simulink model "SigProcessFinished"  (R2022b)
settings: configuration reference "TmVcThermal_Configuration_sub" (kept outside this file)
undefined symbols (not defined in the file): cClCddAdc_D_u16ADNum, cClCddAdc_D_u8FilterType, cClCddAdc_D_u8RawValueNum
libraries: simulink x23
(part 1 of 2)
settings Model: PacingRate=0.500000  Creator=blue.ge  LastModifiedBy=blue.ge
settings ConfigSetRef: SourceName=TmVcThermal_Configuration_sub  SourceLocation=Base Workspace

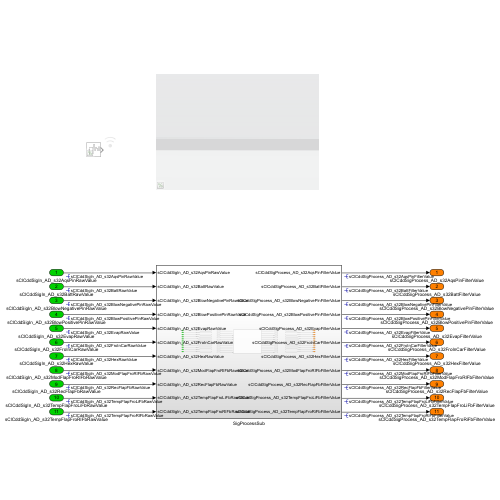
[thumbnail: Simulink's stored preview of the top-level diagram]
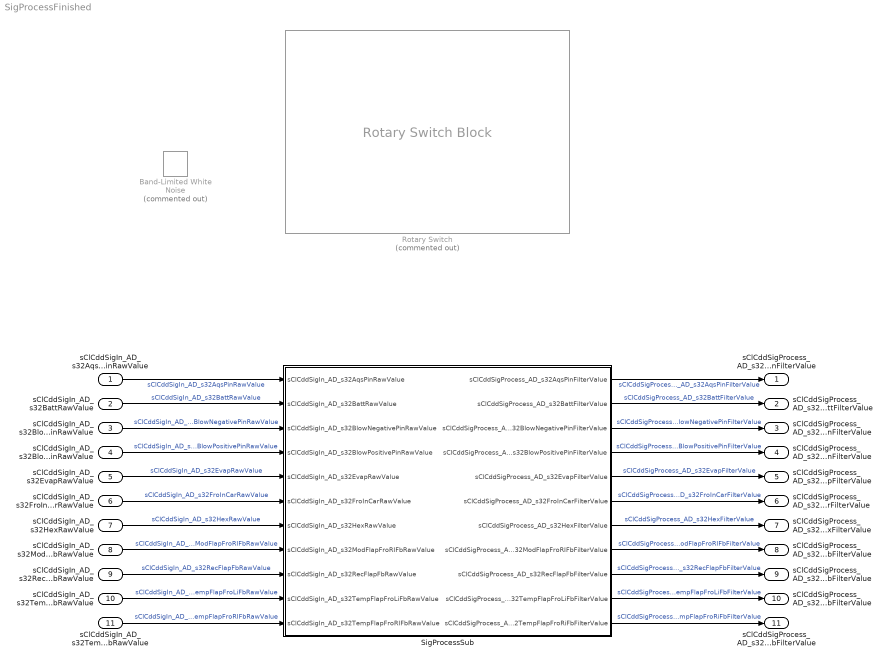
== system SigProcessFinished ==
  sClCddSigIn_AD_s32AqsPinRawValue : Inport  OutDataTypeStr=single
  sClCddSigIn_AD_s32BattRawValue : Inport  Port=2  OutDataTypeStr=single
  sClCddSigIn_AD_s32BlowNegativePinRawValue : Inport  Port=3  OutDataTypeStr=single
  sClCddSigIn_AD_s32BlowPositivePinRawValue : Inport  Port=4  OutDataTypeStr=single
  sClCddSigIn_AD_s32EvapRawValue : Inport  Port=5  OutDataTypeStr=single
  sClCddSigIn_AD_s32FroInCarRawValue : Inport  Port=6  OutDataTypeStr=single
  sClCddSigIn_AD_s32HexRawValue : Inport  Port=7  OutDataTypeStr=single
  sClCddSigIn_AD_s32ModFlapFroRIFbRawValue : Inport  Port=8  OutDataTypeStr=single
  sClCddSigIn_AD_s32RecFlapFbRawValue : Inport  Port=9  OutDataTypeStr=single
  sClCddSigIn_AD_s32TempFlapFroLiFbRawValue : Inport  Port=10  OutDataTypeStr=single
  sClCddSigIn_AD_s32TempFlapFroRIFbRawValue : Inport  Port=11  OutDataTypeStr=single
  Band-Limited White Noise : simulink/Sources/Band-Limited White Noise  Commented=on  Cov=[0.1]  Ts=0.1  seed=[23341]
  Rotary Switch : RotarySwitchBlock  Commented=on
      settings: Values={{'No Filter', 'AvgSortMid', 'AvgSortWithoutEdge', 'AvgSimple', 'AvgQuick'}, [0 1 2 3 4]}
  SigProcessSub : Subsystem
  sClCddSigProcess_AD_s32AqsPinFilterValue : Outport  OutDataTypeStr=single
  sClCddSigProcess_AD_s32BattFilterValue : Outport  Port=2  OutDataTypeStr=single
  sClCddSigProcess_AD_s32BlowNegativePinFilterValue : Outport  Port=3  OutDataTypeStr=single
  sClCddSigProcess_AD_s32BlowPositivePinFilterValue : Outport  Port=4  OutDataTypeStr=single
  sClCddSigProcess_AD_s32EvapFilterValue : Outport  Port=5  OutDataTypeStr=single
  sClCddSigProcess_AD_s32FroInCarFilterValue : Outport  Port=6  OutDataTypeStr=single
  sClCddSigProcess_AD_s32HexFilterValue : Outport  Port=7  OutDataTypeStr=single
  sClCddSigProcess_AD_s32ModFlapFroRIFbFilterValue : Outport  Port=8  OutDataTypeStr=single
  sClCddSigProcess_AD_s32RecFlapFbFilterValue : Outport  Port=9  OutDataTypeStr=single
  sClCddSigProcess_AD_s32TempFlapFroLiFbFilterValue : Outport  Port=10  OutDataTypeStr=single
  sClCddSigProcess_AD_s32TempFlapFroRiFbFilterValue : Outport  Port=11  OutDataTypeStr=single
  wires:
  sClCddSigIn_AD_s32AqsPinRawValue/1 -> SigProcessSub/1(sClCddSigIn_AD_s32AqsPinRawValue)  "sClCddSigIn_AD_s32AqsPinRawValue"
  sClCddSigIn_AD_s32BattRawValue/1 -> SigProcessSub/2(sClCddSigIn_AD_s32BattRawValue)  "sClCddSigIn_AD_s32BattRawValue"
  sClCddSigIn_AD_s32BlowNegativePinRawValue/1 -> SigProcessSub/3(sClCddSigIn_AD_s32BlowNegativePinRawValue)  "sClCddSigIn_AD_s32BlowNegativePinRawValue"
  sClCddSigIn_AD_s32BlowPositivePinRawValue/1 -> SigProcessSub/4(sClCddSigIn_AD_s32BlowPositivePinRawValue)  "sClCddSigIn_AD_s32BlowPositivePinRawValue"
  sClCddSigIn_AD_s32EvapRawValue/1 -> SigProcessSub/5(sClCddSigIn_AD_s32EvapRawValue)  "sClCddSigIn_AD_s32EvapRawValue"
  sClCddSigIn_AD_s32FroInCarRawValue/1 -> SigProcessSub/6(sClCddSigIn_AD_s32FroInCarRawValue)  "sClCddSigIn_AD_s32FroInCarRawValue"
  sClCddSigIn_AD_s32HexRawValue/1 -> SigProcessSub/7(sClCddSigIn_AD_s32HexRawValue)  "sClCddSigIn_AD_s32HexRawValue"
  sClCddSigIn_AD_s32ModFlapFroRIFbRawValue/1 -> SigProcessSub/8(sClCddSigIn_AD_s32ModFlapFroRIFbRawValue)  "sClCddSigIn_AD_s32ModFlapFroRIFbRawValue"
  sClCddSigIn_AD_s32RecFlapFbRawValue/1 -> SigProcessSub/9(sClCddSigIn_AD_s32RecFlapFbRawValue)  "sClCddSigIn_AD_s32RecFlapFbRawValue"
  sClCddSigIn_AD_s32TempFlapFroLiFbRawValue/1 -> SigProcessSub/10(sClCddSigIn_AD_s32TempFlapFroLiFbRawValue)  "sClCddSigIn_AD_s32TempFlapFroLiFbRawValue"
  sClCddSigIn_AD_s32TempFlapFroRIFbRawValue/1 -> SigProcessSub/11(sClCddSigIn_AD_s32TempFlapFroRIFbRawValue)  "sClCddSigIn_AD_s32TempFlapFroRIFbRawValue"
  SigProcessSub/1(sClCddSigProcess_AD_s32AqsPinFilterValue) -> sClCddSigProcess_AD_s32AqsPinFilterValue/1  "sClCddSigProcess_AD_s32AqsPinFilterValue"
  SigProcessSub/2(sClCddSigProcess_AD_s32BattFilterValue) -> sClCddSigProcess_AD_s32BattFilterValue/1  "sClCddSigProcess_AD_s32BattFilterValue"
  SigProcessSub/3(sClCddSigProcess_AD_s32BlowNegativePinFilterValue) -> sClCddSigProcess_AD_s32BlowNegativePinFilterValue/1  "sClCddSigProcess_AD_s32BlowNegativePinFilterValue"
  SigProcessSub/4(sClCddSigProcess_AD_s32BlowPositivePinFilterValue) -> sClCddSigProcess_AD_s32BlowPositivePinFilterValue/1  "sClCddSigProcess_AD_s32BlowPositivePinFilterValue"
  SigProcessSub/5(sClCddSigProcess_AD_s32EvapFilterValue) -> sClCddSigProcess_AD_s32EvapFilterValue/1  "sClCddSigProcess_AD_s32EvapFilterValue"
  SigProcessSub/6(sClCddSigProcess_AD_s32FroInCarFilterValue) -> sClCddSigProcess_AD_s32FroInCarFilterValue/1  "sClCddSigProcess_AD_s32FroInCarFilterValue"
  SigProcessSub/7(sClCddSigProcess_AD_s32HexFilterValue) -> sClCddSigProcess_AD_s32HexFilterValue/1  "sClCddSigProcess_AD_s32HexFilterValue"
  SigProcessSub/8(sClCddSigProcess_AD_s32ModFlapFroRIFbFilterValue) -> sClCddSigProcess_AD_s32ModFlapFroRIFbFilterValue/1  "sClCddSigProcess_AD_s32ModFlapFroRIFbFilterValue"
  SigProcessSub/9(sClCddSigProcess_AD_s32RecFlapFbFilterValue) -> sClCddSigProcess_AD_s32RecFlapFbFilterValue/1  "sClCddSigProcess_AD_s32RecFlapFbFilterValue"
  SigProcessSub/10(sClCddSigProcess_AD_s32TempFlapFroLiFbFilterValue) -> sClCddSigProcess_AD_s32TempFlapFroLiFbFilterValue/1  "sClCddSigProcess_AD_s32TempFlapFroLiFbFilterValue"
  SigProcessSub/11(sClCddSigProcess_AD_s32TempFlapFroRiFbFilterValue) -> sClCddSigProcess_AD_s32TempFlapFroRiFbFilterValue/1  "sClCddSigProcess_AD_s32TempFlapFroRiFbFilterValue"

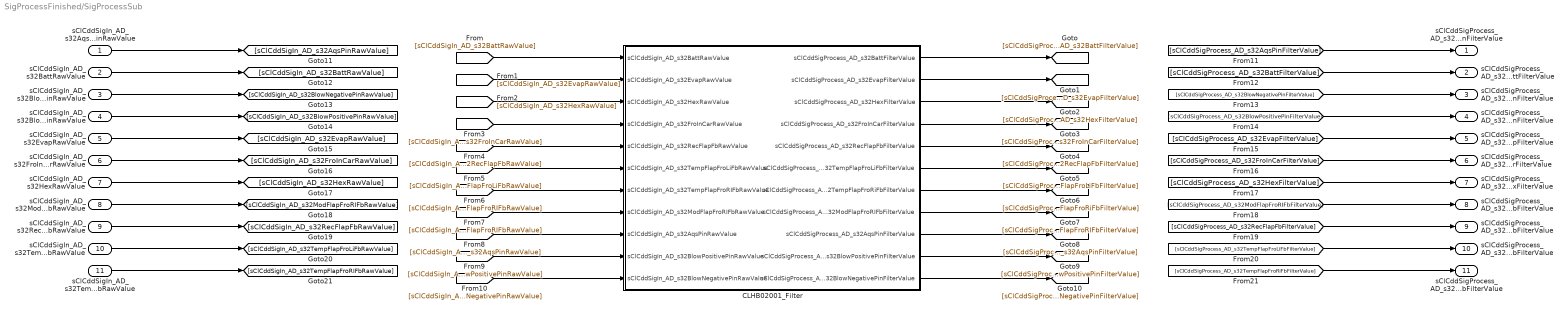
== system SigProcessFinished/SigProcessSub ==
  sClCddSigIn_AD_s32AqsPinRawValue : Inport  OutDataTypeStr=single
  sClCddSigIn_AD_s32BattRawValue : Inport  Port=2  OutDataTypeStr=single
  sClCddSigIn_AD_s32BlowNegativePinRawValue : Inport  Port=3  OutDataTypeStr=single
  sClCddSigIn_AD_s32BlowPositivePinRawValue : Inport  Port=4  OutDataTypeStr=single
  sClCddSigIn_AD_s32EvapRawValue : Inport  Port=5  OutDataTypeStr=single
  sClCddSigIn_AD_s32FroInCarRawValue : Inport  Port=6  OutDataTypeStr=single
  sClCddSigIn_AD_s32HexRawValue : Inport  Port=7  OutDataTypeStr=single
  sClCddSigIn_AD_s32ModFlapFroRIFbRawValue : Inport  Port=8  OutDataTypeStr=single
  sClCddSigIn_AD_s32RecFlapFbRawValue : Inport  Port=9  OutDataTypeStr=single
  sClCddSigIn_AD_s32TempFlapFroLiFbRawValue : Inport  Port=10  OutDataTypeStr=single
  sClCddSigIn_AD_s32TempFlapFroRIFbRawValue : Inport  Port=11  OutDataTypeStr=single
  CLHB02001_Filter : Subsystem
  sClCddSigProcess_AD_s32AqsPinFilterValue : Outport  OutDataTypeStr=single
  sClCddSigProcess_AD_s32BattFilterValue : Outport  Port=2  OutDataTypeStr=single
  sClCddSigProcess_AD_s32BlowNegativePinFilterValue : Outport  Port=3  OutDataTypeStr=single
  sClCddSigProcess_AD_s32BlowPositivePinFilterValue : Outport  Port=4  OutDataTypeStr=single
  sClCddSigProcess_AD_s32EvapFilterValue : Outport  Port=5  OutDataTypeStr=single
  sClCddSigProcess_AD_s32FroInCarFilterValue : Outport  Port=6  OutDataTypeStr=single
  sClCddSigProcess_AD_s32HexFilterValue : Outport  Port=7  OutDataTypeStr=single
  sClCddSigProcess_AD_s32ModFlapFroRIFbFilterValue : Outport  Port=8  OutDataTypeStr=single
  sClCddSigProcess_AD_s32RecFlapFbFilterValue : Outport  Port=9  OutDataTypeStr=single
  sClCddSigProcess_AD_s32TempFlapFroLiFbFilterValue : Outport  Port=10  OutDataTypeStr=single
  sClCddSigProcess_AD_s32TempFlapFroRiFbFilterValue : Outport  Port=11  OutDataTypeStr=single
  wires:
  [sClCddSigIn_AD_s32BattRawValue] -> CLHB02001_Filter/1(sClCddSigIn_AD_s32BattRawValue)
  [sClCddSigIn_AD_s32EvapRawValue] -> CLHB02001_Filter/2(sClCddSigIn_AD_s32EvapRawValue)
  [sClCddSigIn_AD_s32HexRawValue] -> CLHB02001_Filter/3(sClCddSigIn_AD_s32HexRawValue)
  [sClCddSigIn_AD_s32FroInCarRawValue] -> CLHB02001_Filter/4(sClCddSigIn_AD_s32FroInCarRawValue)
  [sClCddSigIn_AD_s32RecFlapFbRawValue] -> CLHB02001_Filter/5(sClCddSigIn_AD_s32RecFlapFbRawValue)
  [sClCddSigIn_AD_s32TempFlapFroLiFbRawValue] -> CLHB02001_Filter/6(sClCddSigIn_AD_s32TempFlapFroLiFbRawValue)
  [sClCddSigIn_AD_s32TempFlapFroRIFbRawValue] -> CLHB02001_Filter/7(sClCddSigIn_AD_s32TempFlapFroRIFbRawValue)
  [sClCddSigIn_AD_s32ModFlapFroRIFbRawValue] -> CLHB02001_Filter/8(sClCddSigIn_AD_s32ModFlapFroRIFbRawValue)
  [sClCddSigIn_AD_s32AqsPinRawValue] -> CLHB02001_Filter/9(sClCddSigIn_AD_s32AqsPinRawValue)
  [sClCddSigIn_AD_s32BlowPositivePinRawValue] -> CLHB02001_Filter/10(sClCddSigIn_AD_s32BlowPositivePinRawValue)
  [sClCddSigIn_AD_s32BlowNegativePinRawValue] -> CLHB02001_Filter/11(sClCddSigIn_AD_s32BlowNegativePinRawValue)
  CLHB02001_Filter/1(sClCddSigProcess_AD_s32BattFilterValue) -> [sClCddSigProcess_AD_s32BattFilterValue]
  CLHB02001_Filter/2(sClCddSigProcess_AD_s32EvapFilterValue) -> [sClCddSigProcess_AD_s32EvapFilterValue]
  CLHB02001_Filter/3(sClCddSigProcess_AD_s32HexFilterValue) -> [sClCddSigProcess_AD_s32HexFilterValue]
  CLHB02001_Filter/4(sClCddSigProcess_AD_s32FroInCarFilterValue) -> [sClCddSigProcess_AD_s32FroInCarFilterValue]
  CLHB02001_Filter/5(sClCddSigProcess_AD_s32RecFlapFbFilterValue) -> [sClCddSigProcess_AD_s32RecFlapFbFilterValue]
  CLHB02001_Filter/6(sClCddSigProcess_AD_s32TempFlapFroLiFbFilterValue) -> [sClCddSigProcess_AD_s32TempFlapFroLiFbFilterValue]
  CLHB02001_Filter/7(sClCddSigProcess_AD_s32TempFlapFroRiFbFilterValue) -> [sClCddSigProcess_AD_s32TempFlapFroRiFbFilterValue]
  CLHB02001_Filter/8(sClCddSigProcess_AD_s32ModFlapFroRIFbFilterValue) -> [sClCddSigProcess_AD_s32ModFlapFroRIFbFilterValue]
  CLHB02001_Filter/9(sClCddSigProcess_AD_s32AqsPinFilterValue) -> [sClCddSigProcess_AD_s32AqsPinFilterValue]
  CLHB02001_Filter/10(sClCddSigProcess_AD_s32BlowPositivePinFilterValue) -> [sClCddSigProcess_AD_s32BlowPositivePinFilterValue]
  CLHB02001_Filter/11(sClCddSigProcess_AD_s32BlowNegativePinFilterValue) -> [sClCddSigProcess_AD_s32BlowNegativePinFilterValue]
  sClCddSigIn_AD_s32AqsPinRawValue/1 -> [sClCddSigIn_AD_s32AqsPinRawValue]
  sClCddSigIn_AD_s32BattRawValue/1 -> [sClCddSigIn_AD_s32BattRawValue]
  sClCddSigIn_AD_s32BlowNegativePinRawValue/1 -> [sClCddSigIn_AD_s32BlowNegativePinRawValue]
  sClCddSigIn_AD_s32BlowPositivePinRawValue/1 -> [sClCddSigIn_AD_s32BlowPositivePinRawValue]
  sClCddSigIn_AD_s32EvapRawValue/1 -> [sClCddSigIn_AD_s32EvapRawValue]
  sClCddSigIn_AD_s32FroInCarRawValue/1 -> [sClCddSigIn_AD_s32FroInCarRawValue]
  sClCddSigIn_AD_s32HexRawValue/1 -> [sClCddSigIn_AD_s32HexRawValue]
  sClCddSigIn_AD_s32ModFlapFroRIFbRawValue/1 -> [sClCddSigIn_AD_s32ModFlapFroRIFbRawValue]
  sClCddSigIn_AD_s32RecFlapFbRawValue/1 -> [sClCddSigIn_AD_s32RecFlapFbRawValue]
  sClCddSigIn_AD_s32TempFlapFroLiFbRawValue/1 -> [sClCddSigIn_AD_s32TempFlapFroLiFbRawValue]
  sClCddSigIn_AD_s32TempFlapFroRIFbRawValue/1 -> [sClCddSigIn_AD_s32TempFlapFroRIFbRawValue]
  [sClCddSigProcess_AD_s32AqsPinFilterValue] -> sClCddSigProcess_AD_s32AqsPinFilterValue/1
  [sClCddSigProcess_AD_s32BattFilterValue] -> sClCddSigProcess_AD_s32BattFilterValue/1
  [sClCddSigProcess_AD_s32BlowNegativePinFilterValue] -> sClCddSigProcess_AD_s32BlowNegativePinFilterValue/1
  [sClCddSigProcess_AD_s32BlowPositivePinFilterValue] -> sClCddSigProcess_AD_s32BlowPositivePinFilterValue/1
  [sClCddSigProcess_AD_s32EvapFilterValue] -> sClCddSigProcess_AD_s32EvapFilterValue/1
  [sClCddSigProcess_AD_s32FroInCarFilterValue] -> sClCddSigProcess_AD_s32FroInCarFilterValue/1
  [sClCddSigProcess_AD_s32HexFilterValue] -> sClCddSigProcess_AD_s32HexFilterValue/1
  [sClCddSigProcess_AD_s32ModFlapFroRIFbFilterValue] -> sClCddSigProcess_AD_s32ModFlapFroRIFbFilterValue/1
  [sClCddSigProcess_AD_s32RecFlapFbFilterValue] -> sClCddSigProcess_AD_s32RecFlapFbFilterValue/1
  [sClCddSigProcess_AD_s32TempFlapFroLiFbFilterValue] -> sClCddSigProcess_AD_s32TempFlapFroLiFbFilterValue/1
  [sClCddSigProcess_AD_s32TempFlapFroRiFbFilterValue] -> sClCddSigProcess_AD_s32TempFlapFroRiFbFilterValue/1

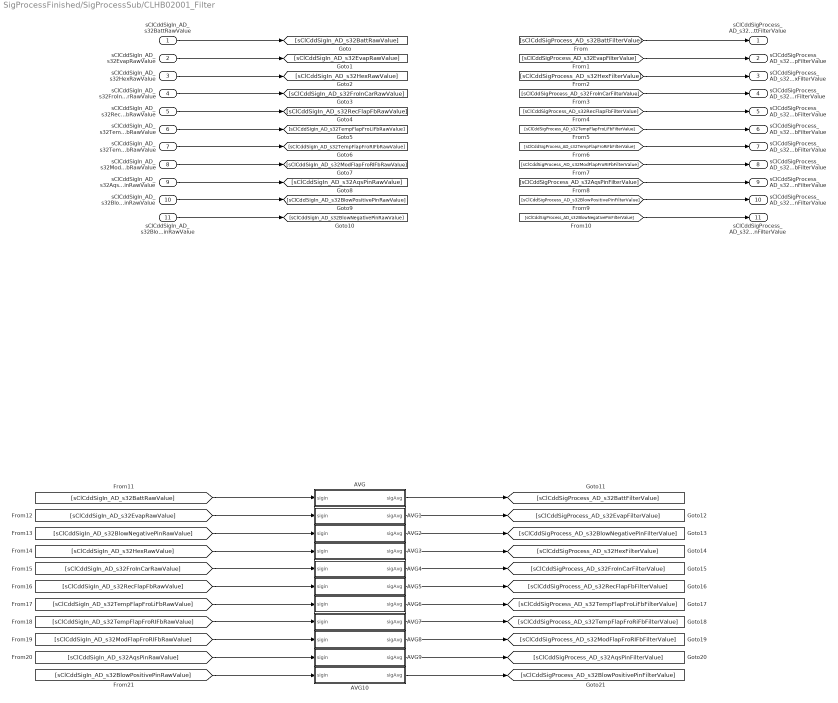
== system SigProcessFinished/SigProcessSub/CLHB02001_Filter ==
  sClCddSigIn_AD_s32BattRawValue : Inport  OutDataTypeStr=single
  sClCddSigIn_AD_s32EvapRawValue : Inport  Port=2  OutDataTypeStr=single
  sClCddSigIn_AD_s32HexRawValue : Inport  Port=3  OutDataTypeStr=single
  sClCddSigIn_AD_s32FroInCarRawValue : Inport  Port=4  OutDataTypeStr=single
  sClCddSigIn_AD_s32RecFlapFbRawValue : Inport  Port=5  OutDataTypeStr=single
  sClCddSigIn_AD_s32TempFlapFroLiFbRawValue : Inport  Port=6  OutDataTypeStr=single
  sClCddSigIn_AD_s32TempFlapFroRIFbRawValue : Inport  Port=7  OutDataTypeStr=single
  sClCddSigIn_AD_s32ModFlapFroRIFbRawValue : Inport  Port=8  OutDataTypeStr=single
  sClCddSigIn_AD_s32AqsPinRawValue : Inport  Port=9  OutDataTypeStr=single
  sClCddSigIn_AD_s32BlowPositivePinRawValue : Inport  Port=10  OutDataTypeStr=single
  sClCddSigIn_AD_s32BlowNegativePinRawValue : Inport  Port=11  OutDataTypeStr=single
  AVG : Subsystem
  AVG1 : Subsystem
  AVG10 : Subsystem
  AVG2 : Subsystem
  AVG3 : Subsystem
  AVG4 : Subsystem
  AVG5 : Subsystem
  AVG6 : Subsystem
  AVG7 : Subsystem
  AVG8 : Subsystem
  AVG9 : Subsystem
  sClCddSigProcess_AD_s32BattFilterValue : Outport  OutDataTypeStr=single
  sClCddSigProcess_AD_s32EvapFilterValue : Outport  Port=2  OutDataTypeStr=single
  sClCddSigProcess_AD_s32HexFilterValue : Outport  Port=3  OutDataTypeStr=single
  sClCddSigProcess_AD_s32FroInCarFilterValue : Outport  Port=4  OutDataTypeStr=single
  sClCddSigProcess_AD_s32RecFlapFbFilterValue : Outport  Port=5  OutDataTypeStr=single
  sClCddSigProcess_AD_s32TempFlapFroLiFbFilterValue : Outport  Port=6  OutDataTypeStr=single
  sClCddSigProcess_AD_s32TempFlapFroRiFbFilterValue : Outport  Port=7  OutDataTypeStr=single
  sClCddSigProcess_AD_s32ModFlapFroRIFbFilterValue : Outport  Port=8  OutDataTypeStr=single
  sClCddSigProcess_AD_s32AqsPinFilterValue : Outport  Port=9  OutDataTypeStr=single
  sClCddSigProcess_AD_s32BlowPositivePinFilterValue : Outport  Port=10  OutDataTypeStr=single
  sClCddSigProcess_AD_s32BlowNegativePinFilterValue : Outport  Port=11  OutDataTypeStr=single
  wires:
  sClCddSigIn_AD_s32BattRawValue/1 -> [sClCddSigIn_AD_s32BattRawValue]
  sClCddSigIn_AD_s32EvapRawValue/1 -> [sClCddSigIn_AD_s32EvapRawValue]
  sClCddSigIn_AD_s32HexRawValue/1 -> [sClCddSigIn_AD_s32HexRawValue]
  sClCddSigIn_AD_s32FroInCarRawValue/1 -> [sClCddSigIn_AD_s32FroInCarRawValue]
  sClCddSigIn_AD_s32RecFlapFbRawValue/1 -> [sClCddSigIn_AD_s32RecFlapFbRawValue]
  sClCddSigIn_AD_s32TempFlapFroLiFbRawValue/1 -> [sClCddSigIn_AD_s32TempFlapFroLiFbRawValue]
  sClCddSigIn_AD_s32TempFlapFroRIFbRawValue/1 -> [sClCddSigIn_AD_s32TempFlapFroRIFbRawValue]
  sClCddSigIn_AD_s32ModFlapFroRIFbRawValue/1 -> [sClCddSigIn_AD_s32ModFlapFroRIFbRawValue]
  sClCddSigIn_AD_s32AqsPinRawValue/1 -> [sClCddSigIn_AD_s32AqsPinRawValue]
  sClCddSigIn_AD_s32BlowPositivePinRawValue/1 -> [sClCddSigIn_AD_s32BlowPositivePinRawValue]
  sClCddSigIn_AD_s32BlowNegativePinRawValue/1 -> [sClCddSigIn_AD_s32BlowNegativePinRawValue]
  [sClCddSigProcess_AD_s32BattFilterValue] -> sClCddSigProcess_AD_s32BattFilterValue/1
  [sClCddSigProcess_AD_s32EvapFilterValue] -> sClCddSigProcess_AD_s32EvapFilterValue/1
  [sClCddSigProcess_AD_s32HexFilterValue] -> sClCddSigProcess_AD_s32HexFilterValue/1
  [sClCddSigProcess_AD_s32FroInCarFilterValue] -> sClCddSigProcess_AD_s32FroInCarFilterValue/1
  [sClCddSigProcess_AD_s32RecFlapFbFilterValue] -> sClCddSigProcess_AD_s32RecFlapFbFilterValue/1
  [sClCddSigProcess_AD_s32TempFlapFroLiFbFilterValue] -> sClCddSigProcess_AD_s32TempFlapFroLiFbFilterValue/1
  [sClCddSigProcess_AD_s32TempFlapFroRiFbFilterValue] -> sClCddSigProcess_AD_s32TempFlapFroRiFbFilterValue/1
  [sClCddSigProcess_AD_s32ModFlapFroRIFbFilterValue] -> sClCddSigProcess_AD_s32ModFlapFroRIFbFilterValue/1
  [sClCddSigProcess_AD_s32AqsPinFilterValue] -> sClCddSigProcess_AD_s32AqsPinFilterValue/1
  [sClCddSigProcess_AD_s32BlowPositivePinFilterValue] -> sClCddSigProcess_AD_s32BlowPositivePinFilterValue/1
  [sClCddSigProcess_AD_s32BlowNegativePinFilterValue] -> sClCddSigProcess_AD_s32BlowNegativePinFilterValue/1
  [sClCddSigIn_AD_s32BattRawValue] -> AVG/1(sigin)
  AVG/1(sigAvg) -> [sClCddSigProcess_AD_s32BattFilterValue]
  [sClCddSigIn_AD_s32EvapRawValue] -> AVG1/1(sigin)
  [sClCddSigIn_AD_s32BlowNegativePinRawValue] -> AVG2/1(sigin)
  [sClCddSigIn_AD_s32HexRawValue] -> AVG3/1(sigin)
  [sClCddSigIn_AD_s32FroInCarRawValue] -> AVG4/1(sigin)
  [sClCddSigIn_AD_s32RecFlapFbRawValue] -> AVG5/1(sigin)
  [sClCddSigIn_AD_s32TempFlapFroLiFbRawValue] -> AVG6/1(sigin)
  [sClCddSigIn_AD_s32TempFlapFroRIFbRawValue] -> AVG7/1(sigin)
  [sClCddSigIn_AD_s32ModFlapFroRIFbRawValue] -> AVG8/1(sigin)
  [sClCddSigIn_AD_s32AqsPinRawValue] -> AVG9/1(sigin)
  [sClCddSigIn_AD_s32BlowPositivePinRawValue] -> AVG10/1(sigin)
  AVG1/1(sigAvg) -> [sClCddSigProcess_AD_s32EvapFilterValue]
  AVG2/1(sigAvg) -> [sClCddSigProcess_AD_s32BlowNegativePinFilterValue]
  AVG3/1(sigAvg) -> [sClCddSigProcess_AD_s32HexFilterValue]
  AVG4/1(sigAvg) -> [sClCddSigProcess_AD_s32FroInCarFilterValue]
  AVG5/1(sigAvg) -> [sClCddSigProcess_AD_s32RecFlapFbFilterValue]
  AVG6/1(sigAvg) -> [sClCddSigProcess_AD_s32TempFlapFroLiFbFilterValue]
  AVG7/1(sigAvg) -> [sClCddSigProcess_AD_s32TempFlapFroRiFbFilterValue]
  AVG8/1(sigAvg) -> [sClCddSigProcess_AD_s32ModFlapFroRIFbFilterValue]
  AVG9/1(sigAvg) -> [sClCddSigProcess_AD_s32AqsPinFilterValue]
  AVG10/1(sigAvg) -> [sClCddSigProcess_AD_s32BlowPositivePinFilterValue]

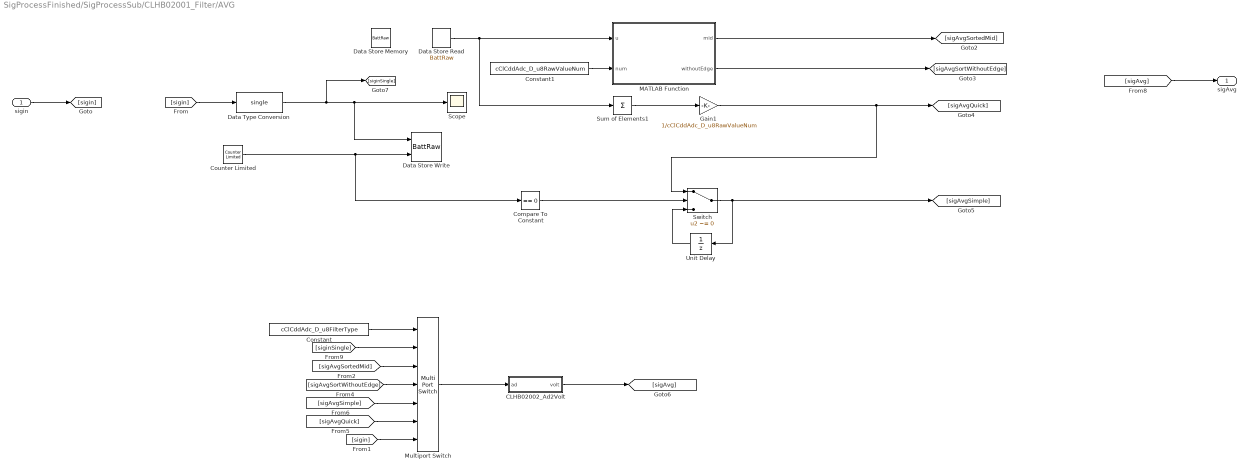
== system SigProcessFinished/SigProcessSub/CLHB02001_Filter/AVG ==
  sigin : Inport
  CLHB02002_Ad2Volt : Subsystem
  Compare To Constant : simulink/Logic and Bit Operations/Compare To Constant  relop===  const=0  OutDataTypeStr=boolean
  Constant : Constant  Value=cClCddAdc_D_u8FilterType  OutDataTypeStr=uint8
  Constant1 : Constant  Value=cClCddAdc_D_u8RawValueNum  OutDataTypeStr=uint8
  Counter Limited : simulink/Sources/Counter Limited  uplimit=cClCddAdc_D_u8RawValueNum-1  tsamp=-1
  Data Store Memory : DataStoreMemory  DataStoreName=BattRaw  ReadBeforeWriteMsg=warning  WriteAfterWriteMsg=warning  WriteAfterReadMsg=warning  ShowAdditionalParam=off  OutDataTypeStr=single  Dimensions=[1 20]
      settings: CopyFcn=set_param(gcbh,'ShowName','off');
  Data Store Read : DataStoreRead  DataStoreName=BattRaw  IndexOptions=Index vector (dialog)  Indices=1  OutputSizes=1
  Data Store Write : DataStoreWrite  DataStoreName=BattRaw  DataStoreElements=BattRaw  EnableIndexing=on  IndexMode=Zero-based  IndexOptions=Index vector (port)  Indices=1  OutputSizes=1
  Data Type Conversion : DataTypeConversion  OutDataTypeStr=single  SaturateOnIntegerOverflow=off  RndMeth=Floor
  Gain1 : Gain  Gain=1/cClCddAdc_D_u8RawValueNum
  MATLAB Function : MATLAB Function  TreatAsAtomicUnit=on
  Multiport Switch : MultiPortSwitch  DataPortOrder=Zero-based contiguous  Inputs=5  DataPortForDefault=Additional data port  zeroidx=on  OutDataTypeStr=single  SaturateOnIntegerOverflow=off  InputSameDT=off
  Scope : Scope
  Sum of Elements1 : Sum  Inputs=+
  Switch : Switch  Criteria=u2 ~= 0  SaturateOnIntegerOverflow=off  InputSameDT=off
  Unit Delay : UnitDelay  SampleTime=-1  HasFrameUpgradeWarning=on
  sigAvg : Outport  OutDataTypeStr=single
  wires:
  Data Store Read/1 -> MATLAB Function/1(u), Sum of Elements1/1
  Sum of Elements1/1 -> Gain1/1
  Compare To Constant/1 -> Switch/2
  Switch/1 -> [sigAvgSimple], Unit Delay/1
  Gain1/1 -> Switch/1, [sigAvgQuick]
  Counter Limited/1 -> Compare To Constant/1, Data Store Write/2
  Data Type Conversion/1 -> [siginSingle], Data Store Write/1, Scope/1
  MATLAB Function/2(withoutEdge) -> [sigAvgSortWithoutEdge]
  Unit Delay/1 -> Switch/3
  MATLAB Function/1(mid) -> [sigAvgSortedMid]
  sigin/1 -> [sigin]
  [sigin] -> Data Type Conversion/1
  [sigin] -> Multiport Switch/7
  Constant/1 -> Multiport Switch/1
  [sigAvgSortedMid] -> Multiport Switch/3
  [sigAvgSortWithoutEdge] -> Multiport Switch/4
  [sigAvgSimple] -> Multiport Switch/5
  [sigAvgQuick] -> Multiport Switch/6
  [siginSingle] -> Multiport Switch/2
  Multiport Switch/1 -> CLHB02002_Ad2Volt/1(ad)
  [sigAvg] -> sigAvg/1
  Constant1/1 -> MATLAB Function/2(num)
  CLHB02002_Ad2Volt/1(volt) -> [sigAvg]

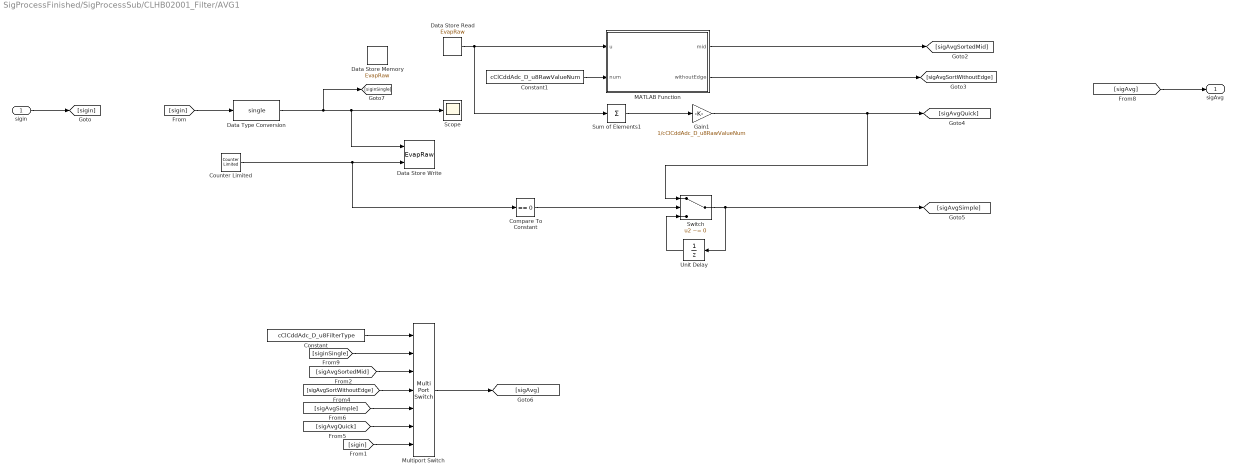
== system SigProcessFinished/SigProcessSub/CLHB02001_Filter/AVG1 ==
  sigin : Inport
  Compare To Constant : simulink/Logic and Bit Operations/Compare To Constant  relop===  const=0  OutDataTypeStr=boolean
  Constant : Constant  Value=cClCddAdc_D_u8FilterType  OutDataTypeStr=uint8
  Constant1 : Constant  Value=cClCddAdc_D_u8RawValueNum  OutDataTypeStr=uint8
  Counter Limited : simulink/Sources/Counter Limited  uplimit=cClCddAdc_D_u8RawValueNum-1  tsamp=-1
  Data Store Memory : DataStoreMemory  DataStoreName=EvapRaw  ReadBeforeWriteMsg=warning  WriteAfterWriteMsg=warning  WriteAfterReadMsg=warning  ShowAdditionalParam=off  OutDataTypeStr=single  Dimensions=[1 20]
      settings: CopyFcn=set_param(gcbh,'ShowName','off');
  Data Store Read : DataStoreRead  DataStoreName=EvapRaw  IndexOptions=Index vector (dialog)  Indices=1  OutputSizes=1
  Data Store Write : DataStoreWrite  DataStoreName=EvapRaw  DataStoreElements=EvapRaw  EnableIndexing=on  IndexMode=Zero-based  IndexOptions=Index vector (port)  Indices=1  OutputSizes=1
  Data Type Conversion : DataTypeConversion  OutDataTypeStr=single  SaturateOnIntegerOverflow=off  RndMeth=Floor
  Gain1 : Gain  Gain=1/cClCddAdc_D_u8RawValueNum
  MATLAB Function : MATLAB Function  TreatAsAtomicUnit=on
  Multiport Switch : MultiPortSwitch  DataPortOrder=Zero-based contiguous  Inputs=5  DataPortForDefault=Additional data port  zeroidx=on  OutDataTypeStr=single  SaturateOnIntegerOverflow=off  InputSameDT=off
  Scope : Scope
  Sum of Elements1 : Sum  Inputs=+
  Switch : Switch  Criteria=u2 ~= 0  SaturateOnIntegerOverflow=off  InputSameDT=off
  Unit Delay : UnitDelay  SampleTime=-1  HasFrameUpgradeWarning=on
  sigAvg : Outport  OutDataTypeStr=single
  wires:
  Constant1/1 -> MATLAB Function/2(num)
  [sigAvg] -> sigAvg/1
  Multiport Switch/1 -> [sigAvg]
  [siginSingle] -> Multiport Switch/2
  [sigAvgQuick] -> Multiport Switch/6
  [sigAvgSimple] -> Multiport Switch/5
  [sigAvgSortWithoutEdge] -> Multiport Switch/4
  [sigAvgSortedMid] -> Multiport Switch/3
  Constant/1 -> Multiport Switch/1
  [sigin] -> Multiport Switch/7
  [sigin] -> Data Type Conversion/1
  sigin/1 -> [sigin]
  MATLAB Function/1(mid) -> [sigAvgSortedMid]
  Unit Delay/1 -> Switch/3
  MATLAB Function/2(withoutEdge) -> [sigAvgSortWithoutEdge]
  Data Type Conversion/1 -> Scope/1, Data Store Write/1, [siginSingle]
  Counter Limited/1 -> Data Store Write/2, Compare To Constant/1
  Gain1/1 -> [sigAvgQuick], Switch/1
  Switch/1 -> Unit Delay/1, [sigAvgSimple]
  Compare To Constant/1 -> Switch/2
  Sum of Elements1/1 -> Gain1/1
  Data Store Read/1 -> Sum of Elements1/1, MATLAB Function/1(u)

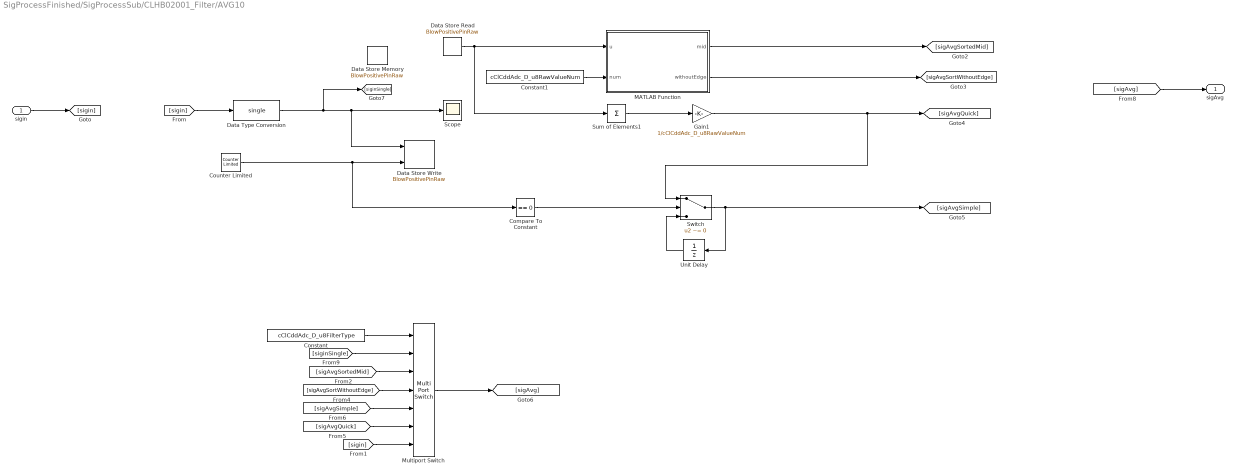
== system SigProcessFinished/SigProcessSub/CLHB02001_Filter/AVG10 ==
  sigin : Inport
  Compare To Constant : simulink/Logic and Bit Operations/Compare To Constant  relop===  const=0  OutDataTypeStr=boolean
  Constant : Constant  Value=cClCddAdc_D_u8FilterType  OutDataTypeStr=uint8
  Constant1 : Constant  Value=cClCddAdc_D_u8RawValueNum  OutDataTypeStr=uint8
  Counter Limited : simulink/Sources/Counter Limited  uplimit=cClCddAdc_D_u8RawValueNum-1  tsamp=-1
  Data Store Memory : DataStoreMemory  DataStoreName=BlowPositivePinRaw  ReadBeforeWriteMsg=warning  WriteAfterWriteMsg=warning  WriteAfterReadMsg=warning  ShowAdditionalParam=off  OutDataTypeStr=single  Dimensions=[1 20]
      settings: CopyFcn=set_param(gcbh,'ShowName','off');
  Data Store Read : DataStoreRead  DataStoreName=BlowPositivePinRaw  IndexOptions=Index vector (dialog)  Indices=1  OutputSizes=1
  Data Store Write : DataStoreWrite  DataStoreName=BlowPositivePinRaw  DataStoreElements=BlowPositivePinRaw  EnableIndexing=on  IndexMode=Zero-based  IndexOptions=Index vector (port)  Indices=1  OutputSizes=1
  Data Type Conversion : DataTypeConversion  OutDataTypeStr=single  SaturateOnIntegerOverflow=off  RndMeth=Floor
  Gain1 : Gain  Gain=1/cClCddAdc_D_u8RawValueNum
  MATLAB Function : MATLAB Function  TreatAsAtomicUnit=on
  Multiport Switch : MultiPortSwitch  DataPortOrder=Zero-based contiguous  Inputs=5  DataPortForDefault=Additional data port  zeroidx=on  OutDataTypeStr=single  SaturateOnIntegerOverflow=off  InputSameDT=off
  Scope : Scope
  Sum of Elements1 : Sum  Inputs=+
  Switch : Switch  Criteria=u2 ~= 0  SaturateOnIntegerOverflow=off  InputSameDT=off
  Unit Delay : UnitDelay  SampleTime=-1  HasFrameUpgradeWarning=on
  sigAvg : Outport  OutDataTypeStr=single
  wires:
  Data Store Read/1 -> MATLAB Function/1(u), Sum of Elements1/1
  Sum of Elements1/1 -> Gain1/1
  Compare To Constant/1 -> Switch/2
  Switch/1 -> [sigAvgSimple], Unit Delay/1
  Gain1/1 -> Switch/1, [sigAvgQuick]
  Counter Limited/1 -> Compare To Constant/1, Data Store Write/2
  Data Type Conversion/1 -> [siginSingle], Data Store Write/1, Scope/1
  MATLAB Function/2(withoutEdge) -> [sigAvgSortWithoutEdge]
  Unit Delay/1 -> Switch/3
  MATLAB Function/1(mid) -> [sigAvgSortedMid]
  sigin/1 -> [sigin]
  [sigin] -> Data Type Conversion/1
  [sigin] -> Multiport Switch/7
  Constant/1 -> Multiport Switch/1
  [sigAvgSortedMid] -> Multiport Switch/3
  [sigAvgSortWithoutEdge] -> Multiport Switch/4
  [sigAvgSimple] -> Multiport Switch/5
  [sigAvgQuick] -> Multiport Switch/6
  [siginSingle] -> Multiport Switch/2
  Multiport Switch/1 -> [sigAvg]
  [sigAvg] -> sigAvg/1
  Constant1/1 -> MATLAB Function/2(num)

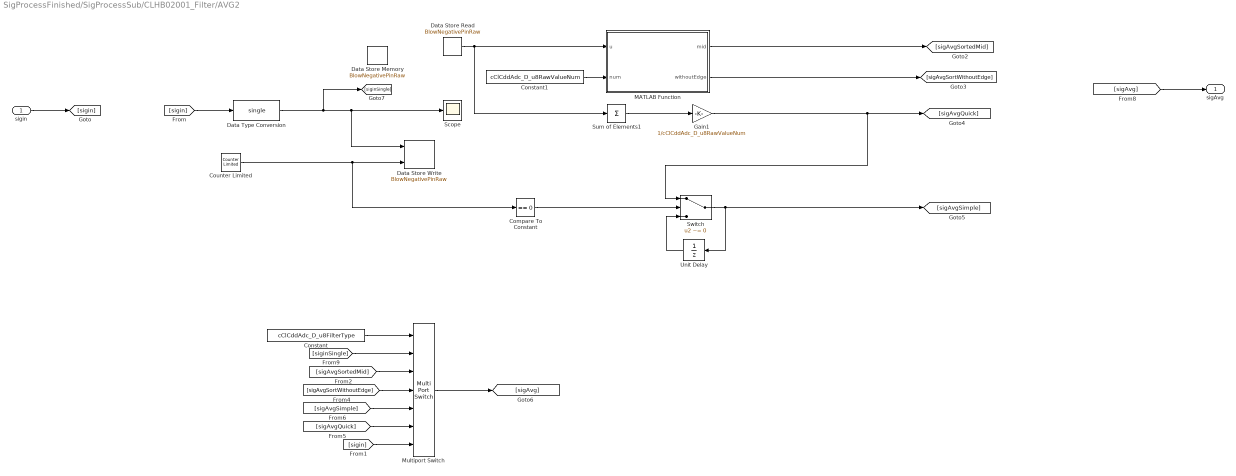
== system SigProcessFinished/SigProcessSub/CLHB02001_Filter/AVG2 ==
  sigin : Inport
  Compare To Constant : simulink/Logic and Bit Operations/Compare To Constant  relop===  const=0  OutDataTypeStr=boolean
  Constant : Constant  Value=cClCddAdc_D_u8FilterType  OutDataTypeStr=uint8
  Constant1 : Constant  Value=cClCddAdc_D_u8RawValueNum  OutDataTypeStr=uint8
  Counter Limited : simulink/Sources/Counter Limited  uplimit=cClCddAdc_D_u8RawValueNum-1  tsamp=-1
  Data Store Memory : DataStoreMemory  DataStoreName=BlowNegativePinRaw  ReadBeforeWriteMsg=warning  WriteAfterWriteMsg=warning  WriteAfterReadMsg=warning  ShowAdditionalParam=off  OutDataTypeStr=single  Dimensions=[1 20]
      settings: CopyFcn=set_param(gcbh,'ShowName','off');
  Data Store Read : DataStoreRead  DataStoreName=BlowNegativePinRaw  IndexOptions=Index vector (dialog)  Indices=1  OutputSizes=1
  Data Store Write : DataStoreWrite  DataStoreName=BlowNegativePinRaw  DataStoreElements=BlowNegativePinRaw  EnableIndexing=on  IndexMode=Zero-based  IndexOptions=Index vector (port)  Indices=1  OutputSizes=1
  Data Type Conversion : DataTypeConversion  OutDataTypeStr=single  SaturateOnIntegerOverflow=off  RndMeth=Floor
  Gain1 : Gain  Gain=1/cClCddAdc_D_u8RawValueNum
  MATLAB Function : MATLAB Function  TreatAsAtomicUnit=on
  Multiport Switch : MultiPortSwitch  DataPortOrder=Zero-based contiguous  Inputs=5  DataPortForDefault=Additional data port  zeroidx=on  OutDataTypeStr=single  SaturateOnIntegerOverflow=off  InputSameDT=off
  Scope : Scope
  Sum of Elements1 : Sum  Inputs=+
  Switch : Switch  Criteria=u2 ~= 0  SaturateOnIntegerOverflow=off  InputSameDT=off
  Unit Delay : UnitDelay  SampleTime=-1  HasFrameUpgradeWarning=on
  sigAvg : Outport  OutDataTypeStr=single
  wires:
  Data Store Read/1 -> MATLAB Function/1(u), Sum of Elements1/1
  Sum of Elements1/1 -> Gain1/1
  Compare To Constant/1 -> Switch/2
  Switch/1 -> [sigAvgSimple], Unit Delay/1
  Gain1/1 -> Switch/1, [sigAvgQuick]
  Counter Limited/1 -> Compare To Constant/1, Data Store Write/2
  Data Type Conversion/1 -> [siginSingle], Data Store Write/1, Scope/1
  MATLAB Function/2(withoutEdge) -> [sigAvgSortWithoutEdge]
  Unit Delay/1 -> Switch/3
  MATLAB Function/1(mid) -> [sigAvgSortedMid]
  sigin/1 -> [sigin]
  [sigin] -> Data Type Conversion/1
  [sigin] -> Multiport Switch/7
  Constant/1 -> Multiport Switch/1
  [sigAvgSortedMid] -> Multiport Switch/3
  [sigAvgSortWithoutEdge] -> Multiport Switch/4
  [sigAvgSimple] -> Multiport Switch/5
  [sigAvgQuick] -> Multiport Switch/6
  [siginSingle] -> Multiport Switch/2
  Multiport Switch/1 -> [sigAvg]
  [sigAvg] -> sigAvg/1
  Constant1/1 -> MATLAB Function/2(num)

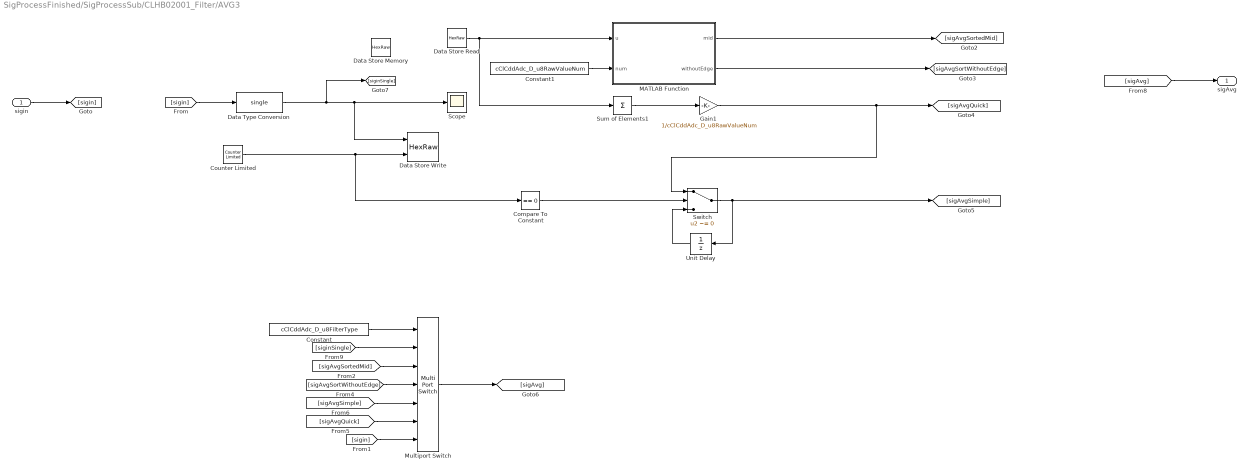
== system SigProcessFinished/SigProcessSub/CLHB02001_Filter/AVG3 ==
  sigin : Inport
  Compare To Constant : simulink/Logic and Bit Operations/Compare To Constant  relop===  const=0  OutDataTypeStr=boolean
  Constant : Constant  Value=cClCddAdc_D_u8FilterType  OutDataTypeStr=uint8
  Constant1 : Constant  Value=cClCddAdc_D_u8RawValueNum  OutDataTypeStr=uint8
  Counter Limited : simulink/Sources/Counter Limited  uplimit=cClCddAdc_D_u8RawValueNum-1  tsamp=-1
  Data Store Memory : DataStoreMemory  DataStoreName=HexRaw  ReadBeforeWriteMsg=warning  WriteAfterWriteMsg=warning  WriteAfterReadMsg=warning  ShowAdditionalParam=off  OutDataTypeStr=single  Dimensions=[1 20]
      settings: CopyFcn=set_param(gcbh,'ShowName','off');
  Data Store Read : DataStoreRead  DataStoreName=HexRaw  IndexOptions=Index vector (dialog)  Indices=1  OutputSizes=1
  Data Store Write : DataStoreWrite  DataStoreName=HexRaw  DataStoreElements=HexRaw  EnableIndexing=on  IndexMode=Zero-based  IndexOptions=Index vector (port)  Indices=1  OutputSizes=1
  Data Type Conversion : DataTypeConversion  OutDataTypeStr=single  SaturateOnIntegerOverflow=off  RndMeth=Floor
  Gain1 : Gain  Gain=1/cClCddAdc_D_u8RawValueNum
  MATLAB Function : MATLAB Function  TreatAsAtomicUnit=on
  Multiport Switch : MultiPortSwitch  DataPortOrder=Zero-based contiguous  Inputs=5  DataPortForDefault=Additional data port  zeroidx=on  OutDataTypeStr=single  SaturateOnIntegerOverflow=off  InputSameDT=off
  Scope : Scope
  Sum of Elements1 : Sum  Inputs=+
  Switch : Switch  Criteria=u2 ~= 0  SaturateOnIntegerOverflow=off  InputSameDT=off
  Unit Delay : UnitDelay  SampleTime=-1  HasFrameUpgradeWarning=on
  sigAvg : Outport  OutDataTypeStr=single
  wires:
  Constant1/1 -> MATLAB Function/2(num)
  [sigAvg] -> sigAvg/1
  Multiport Switch/1 -> [sigAvg]
  [siginSingle] -> Multiport Switch/2
  [sigAvgQuick] -> Multiport Switch/6
  [sigAvgSimple] -> Multiport Switch/5
  [sigAvgSortWithoutEdge] -> Multiport Switch/4
  [sigAvgSortedMid] -> Multiport Switch/3
  Constant/1 -> Multiport Switch/1
  [sigin] -> Multiport Switch/7
  [sigin] -> Data Type Conversion/1
  sigin/1 -> [sigin]
  MATLAB Function/1(mid) -> [sigAvgSortedMid]
  Unit Delay/1 -> Switch/3
  MATLAB Function/2(withoutEdge) -> [sigAvgSortWithoutEdge]
  Data Type Conversion/1 -> Scope/1, Data Store Write/1, [siginSingle]
  Counter Limited/1 -> Data Store Write/2, Compare To Constant/1
  Gain1/1 -> [sigAvgQuick], Switch/1
  Switch/1 -> Unit Delay/1, [sigAvgSimple]
  Compare To Constant/1 -> Switch/2
  Sum of Elements1/1 -> Gain1/1
  Data Store Read/1 -> Sum of Elements1/1, MATLAB Function/1(u)

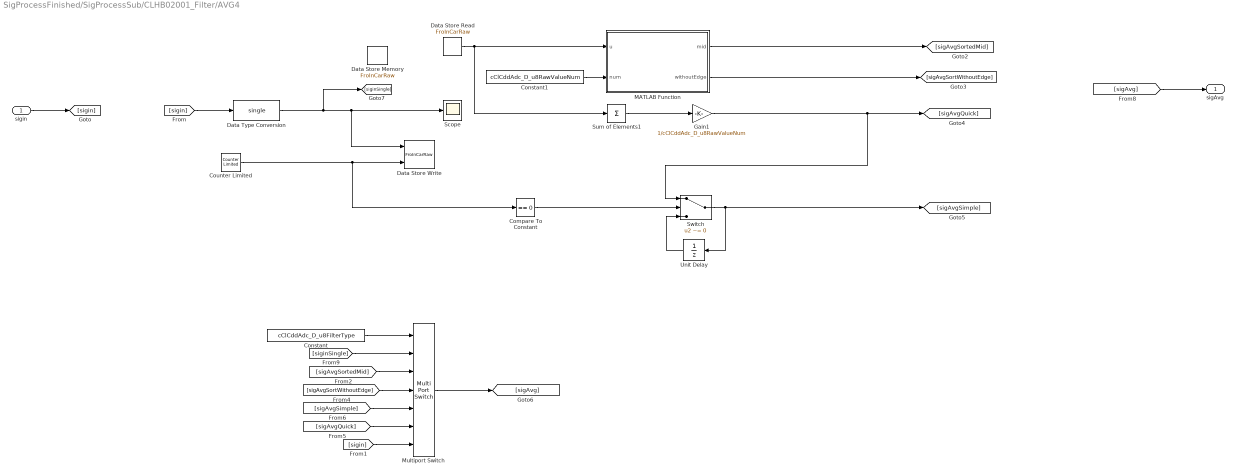
== system SigProcessFinished/SigProcessSub/CLHB02001_Filter/AVG4 ==
  sigin : Inport
  Compare To Constant : simulink/Logic and Bit Operations/Compare To Constant  relop===  const=0  OutDataTypeStr=boolean
  Constant : Constant  Value=cClCddAdc_D_u8FilterType  OutDataTypeStr=uint8
  Constant1 : Constant  Value=cClCddAdc_D_u8RawValueNum  OutDataTypeStr=uint8
  Counter Limited : simulink/Sources/Counter Limited  uplimit=cClCddAdc_D_u8RawValueNum-1  tsamp=-1
  Data Store Memory : DataStoreMemory  DataStoreName=FroInCarRaw  ReadBeforeWriteMsg=warning  WriteAfterWriteMsg=warning  WriteAfterReadMsg=warning  ShowAdditionalParam=off  OutDataTypeStr=single  Dimensions=[1 20]
      settings: CopyFcn=set_param(gcbh,'ShowName','off');
  Data Store Read : DataStoreRead  DataStoreName=FroInCarRaw  IndexOptions=Index vector (dialog)  Indices=1  OutputSizes=1
  Data Store Write : DataStoreWrite  DataStoreName=FroInCarRaw  DataStoreElements=FroInCarRaw  EnableIndexing=on  IndexMode=Zero-based  IndexOptions=Index vector (port)  Indices=1  OutputSizes=1
  Data Type Conversion : DataTypeConversion  OutDataTypeStr=single  SaturateOnIntegerOverflow=off  RndMeth=Floor
  Gain1 : Gain  Gain=1/cClCddAdc_D_u8RawValueNum
  MATLAB Function : MATLAB Function  TreatAsAtomicUnit=on
  Multiport Switch : MultiPortSwitch  DataPortOrder=Zero-based contiguous  Inputs=5  DataPortForDefault=Additional data port  zeroidx=on  OutDataTypeStr=single  SaturateOnIntegerOverflow=off  InputSameDT=off
  Scope : Scope
  Sum of Elements1 : Sum  Inputs=+
  Switch : Switch  Criteria=u2 ~= 0  SaturateOnIntegerOverflow=off  InputSameDT=off
  Unit Delay : UnitDelay  SampleTime=-1  HasFrameUpgradeWarning=on
  sigAvg : Outport  OutDataTypeStr=single
  wires:
  Data Store Read/1 -> MATLAB Function/1(u), Sum of Elements1/1
  Sum of Elements1/1 -> Gain1/1
  Compare To Constant/1 -> Switch/2
  Switch/1 -> [sigAvgSimple], Unit Delay/1
  Gain1/1 -> Switch/1, [sigAvgQuick]
  Counter Limited/1 -> Compare To Constant/1, Data Store Write/2
  Data Type Conversion/1 -> [siginSingle], Data Store Write/1, Scope/1
  MATLAB Function/2(withoutEdge) -> [sigAvgSortWithoutEdge]
  Unit Delay/1 -> Switch/3
  MATLAB Function/1(mid) -> [sigAvgSortedMid]
  sigin/1 -> [sigin]
  [sigin] -> Data Type Conversion/1
  [sigin] -> Multiport Switch/7
  Constant/1 -> Multiport Switch/1
  [sigAvgSortedMid] -> Multiport Switch/3
  [sigAvgSortWithoutEdge] -> Multiport Switch/4
  [sigAvgSimple] -> Multiport Switch/5
  [sigAvgQuick] -> Multiport Switch/6
  [siginSingle] -> Multiport Switch/2
  Multiport Switch/1 -> [sigAvg]
  [sigAvg] -> sigAvg/1
  Constant1/1 -> MATLAB Function/2(num)

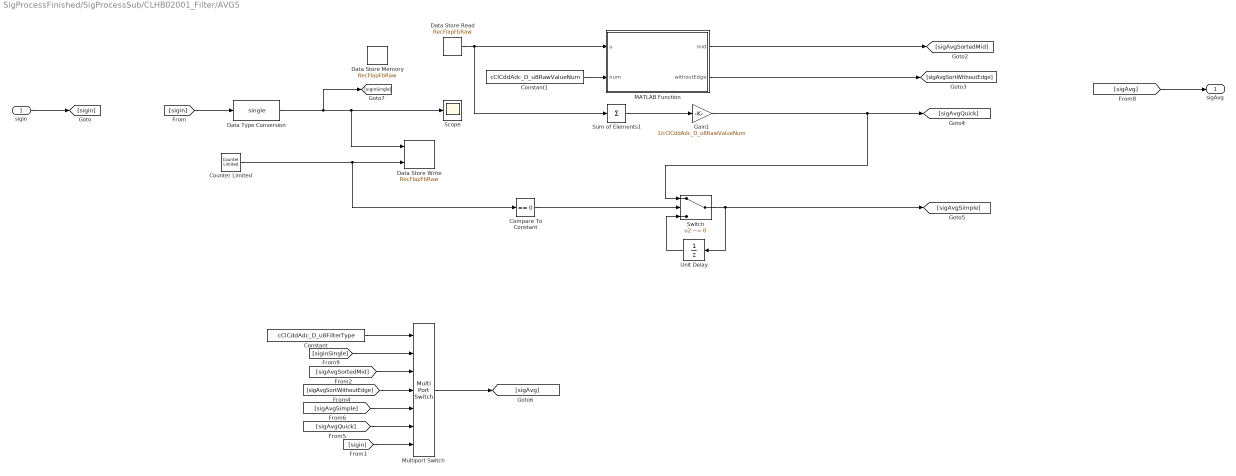
== system SigProcessFinished/SigProcessSub/CLHB02001_Filter/AVG5 ==
  sigin : Inport
  Compare To Constant : simulink/Logic and Bit Operations/Compare To Constant  relop===  const=0  OutDataTypeStr=boolean
  Constant : Constant  Value=cClCddAdc_D_u8FilterType  OutDataTypeStr=uint8
  Constant1 : Constant  Value=cClCddAdc_D_u8RawValueNum  OutDataTypeStr=uint8
  Counter Limited : simulink/Sources/Counter Limited  uplimit=cClCddAdc_D_u8RawValueNum-1  tsamp=-1
  Data Store Memory : DataStoreMemory  DataStoreName=RecFlapFbRaw  ReadBeforeWriteMsg=warning  WriteAfterWriteMsg=warning  WriteAfterReadMsg=warning  ShowAdditionalParam=off  OutDataTypeStr=single  Dimensions=[1 20]
      settings: CopyFcn=set_param(gcbh,'ShowName','off');
  Data Store Read : DataStoreRead  DataStoreName=RecFlapFbRaw  IndexOptions=Index vector (dialog)  Indices=1  OutputSizes=1
  Data Store Write : DataStoreWrite  DataStoreName=RecFlapFbRaw  DataStoreElements=RecFlapFbRaw  EnableIndexing=on  IndexMode=Zero-based  IndexOptions=Index vector (port)  Indices=1  OutputSizes=1
  Data Type Conversion : DataTypeConversion  OutDataTypeStr=single  SaturateOnIntegerOverflow=off  RndMeth=Floor
  Gain1 : Gain  Gain=1/cClCddAdc_D_u8RawValueNum
  MATLAB Function : MATLAB Function  TreatAsAtomicUnit=on
  Multiport Switch : MultiPortSwitch  DataPortOrder=Zero-based contiguous  Inputs=5  DataPortForDefault=Additional data port  zeroidx=on  OutDataTypeStr=single  SaturateOnIntegerOverflow=off  InputSameDT=off
  Scope : Scope
  Sum of Elements1 : Sum  Inputs=+
  Switch : Switch  Criteria=u2 ~= 0  SaturateOnIntegerOverflow=off  InputSameDT=off
  Unit Delay : UnitDelay  SampleTime=-1  HasFrameUpgradeWarning=on
  sigAvg : Outport  OutDataTypeStr=single
  wires:
  Constant1/1 -> MATLAB Function/2(num)
  [sigAvg] -> sigAvg/1
  Multiport Switch/1 -> [sigAvg]
  [siginSingle] -> Multiport Switch/2
  [sigAvgQuick] -> Multiport Switch/6
  [sigAvgSimple] -> Multiport Switch/5
  [sigAvgSortWithoutEdge] -> Multiport Switch/4
  [sigAvgSortedMid] -> Multiport Switch/3
  Constant/1 -> Multiport Switch/1
  [sigin] -> Multiport Switch/7
  [sigin] -> Data Type Conversion/1
  sigin/1 -> [sigin]
  MATLAB Function/1(mid) -> [sigAvgSortedMid]
  Unit Delay/1 -> Switch/3
  MATLAB Function/2(withoutEdge) -> [sigAvgSortWithoutEdge]
  Data Type Conversion/1 -> Scope/1, Data Store Write/1, [siginSingle]
  Counter Limited/1 -> Data Store Write/2, Compare To Constant/1
  Gain1/1 -> [sigAvgQuick], Switch/1
  Switch/1 -> Unit Delay/1, [sigAvgSimple]
  Compare To Constant/1 -> Switch/2
  Sum of Elements1/1 -> Gain1/1
  Data Store Read/1 -> Sum of Elements1/1, MATLAB Function/1(u)

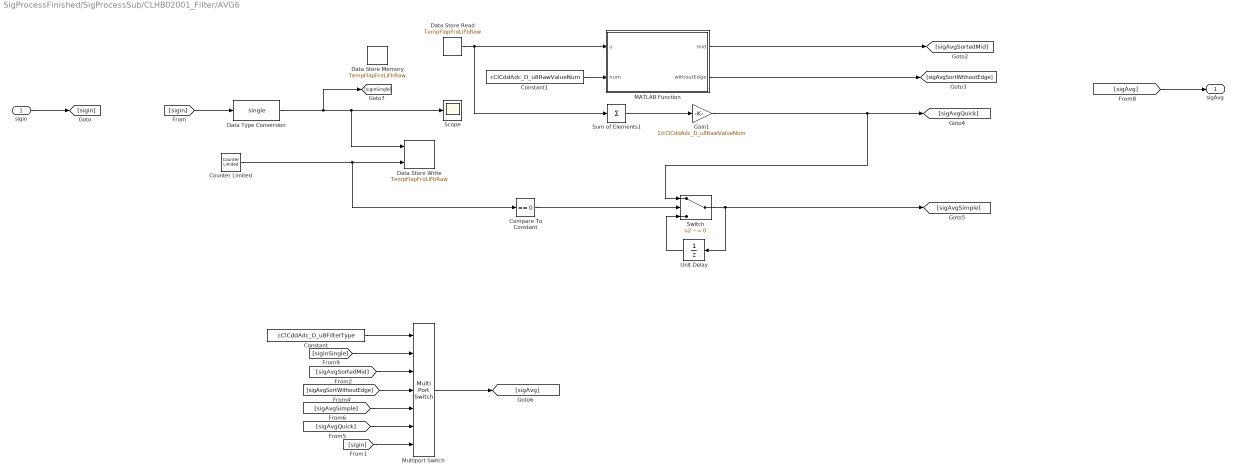
== system SigProcessFinished/SigProcessSub/CLHB02001_Filter/AVG6 ==
  sigin : Inport
  Compare To Constant : simulink/Logic and Bit Operations/Compare To Constant  relop===  const=0  OutDataTypeStr=boolean
  Constant : Constant  Value=cClCddAdc_D_u8FilterType  OutDataTypeStr=uint8
  Constant1 : Constant  Value=cClCddAdc_D_u8RawValueNum  OutDataTypeStr=uint8
  Counter Limited : simulink/Sources/Counter Limited  uplimit=cClCddAdc_D_u8RawValueNum-1  tsamp=-1
  Data Store Memory : DataStoreMemory  DataStoreName=TempFlapFroLiFbRaw  ReadBeforeWriteMsg=warning  WriteAfterWriteMsg=warning  WriteAfterReadMsg=warning  ShowAdditionalParam=off  OutDataTypeStr=single  Dimensions=[1 20]
      settings: CopyFcn=set_param(gcbh,'ShowName','off');
  Data Store Read : DataStoreRead  DataStoreName=TempFlapFroLiFbRaw  IndexOptions=Index vector (dialog)  Indices=1  OutputSizes=1
  Data Store Write : DataStoreWrite  DataStoreName=TempFlapFroLiFbRaw  DataStoreElements=TempFlapFroLiFbRaw  EnableIndexing=on  IndexMode=Zero-based  IndexOptions=Index vector (port)  Indices=1  OutputSizes=1
  Data Type Conversion : DataTypeConversion  OutDataTypeStr=single  SaturateOnIntegerOverflow=off  RndMeth=Floor
  Gain1 : Gain  Gain=1/cClCddAdc_D_u8RawValueNum
  MATLAB Function : MATLAB Function  TreatAsAtomicUnit=on
  Multiport Switch : MultiPortSwitch  DataPortOrder=Zero-based contiguous  Inputs=5  DataPortForDefault=Additional data port  zeroidx=on  OutDataTypeStr=single  SaturateOnIntegerOverflow=off  InputSameDT=off
  Scope : Scope
  Sum of Elements1 : Sum  Inputs=+
  Switch : Switch  Criteria=u2 ~= 0  SaturateOnIntegerOverflow=off  InputSameDT=off
  Unit Delay : UnitDelay  SampleTime=-1  HasFrameUpgradeWarning=on
  sigAvg : Outport  OutDataTypeStr=single
  wires:
  Data Store Read/1 -> MATLAB Function/1(u), Sum of Elements1/1
  Sum of Elements1/1 -> Gain1/1
  Compare To Constant/1 -> Switch/2
  Switch/1 -> [sigAvgSimple], Unit Delay/1
  Gain1/1 -> Switch/1, [sigAvgQuick]
  Counter Limited/1 -> Compare To Constant/1, Data Store Write/2
  Data Type Conversion/1 -> [siginSingle], Data Store Write/1, Scope/1
  MATLAB Function/2(withoutEdge) -> [sigAvgSortWithoutEdge]
  Unit Delay/1 -> Switch/3
  MATLAB Function/1(mid) -> [sigAvgSortedMid]
  sigin/1 -> [sigin]
  [sigin] -> Data Type Conversion/1
  [sigin] -> Multiport Switch/7
  Constant/1 -> Multiport Switch/1
  [sigAvgSortedMid] -> Multiport Switch/3
  [sigAvgSortWithoutEdge] -> Multiport Switch/4
  [sigAvgSimple] -> Multiport Switch/5
  [sigAvgQuick] -> Multiport Switch/6
  [siginSingle] -> Multiport Switch/2
  Multiport Switch/1 -> [sigAvg]
  [sigAvg] -> sigAvg/1
  Constant1/1 -> MATLAB Function/2(num)

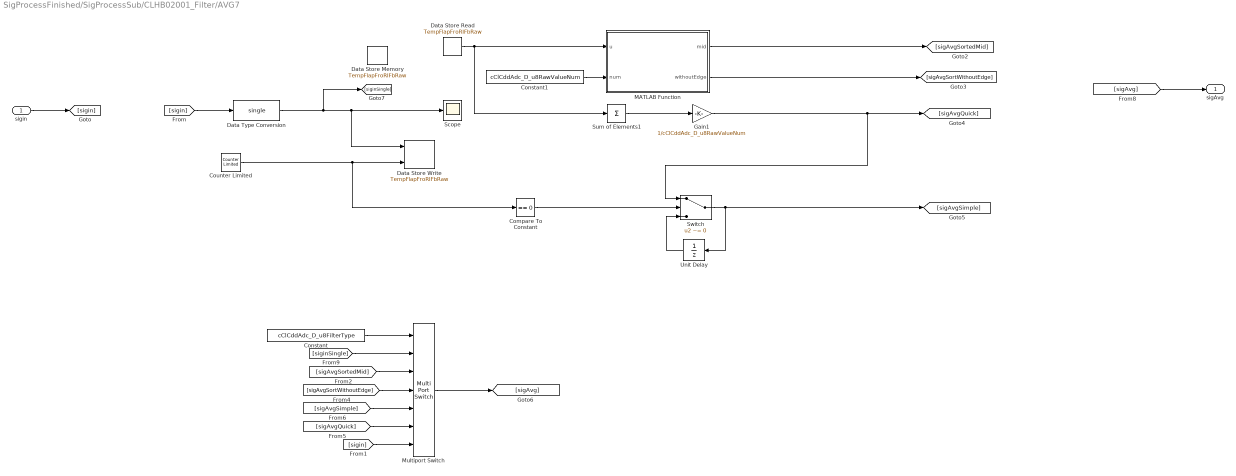
== system SigProcessFinished/SigProcessSub/CLHB02001_Filter/AVG7 ==
  sigin : Inport
  Compare To Constant : simulink/Logic and Bit Operations/Compare To Constant  relop===  const=0  OutDataTypeStr=boolean
  Constant : Constant  Value=cClCddAdc_D_u8FilterType  OutDataTypeStr=uint8
  Constant1 : Constant  Value=cClCddAdc_D_u8RawValueNum  OutDataTypeStr=uint8
  Counter Limited : simulink/Sources/Counter Limited  uplimit=cClCddAdc_D_u8RawValueNum-1  tsamp=-1
  Data Store Memory : DataStoreMemory  DataStoreName=TempFlapFroRIFbRaw  ReadBeforeWriteMsg=warning  WriteAfterWriteMsg=warning  WriteAfterReadMsg=warning  ShowAdditionalParam=off  OutDataTypeStr=single  Dimensions=[1 20]
      settings: CopyFcn=set_param(gcbh,'ShowName','off');
  Data Store Read : DataStoreRead  DataStoreName=TempFlapFroRIFbRaw  IndexOptions=Index vector (dialog)  Indices=1  OutputSizes=1
  Data Store Write : DataStoreWrite  DataStoreName=TempFlapFroRIFbRaw  DataStoreElements=TempFlapFroRIFbRaw  EnableIndexing=on  IndexMode=Zero-based  IndexOptions=Index vector (port)  Indices=1  OutputSizes=1
  Data Type Conversion : DataTypeConversion  OutDataTypeStr=single  SaturateOnIntegerOverflow=off  RndMeth=Floor
  Gain1 : Gain  Gain=1/cClCddAdc_D_u8RawValueNum
  MATLAB Function : MATLAB Function  TreatAsAtomicUnit=on
  Multiport Switch : MultiPortSwitch  DataPortOrder=Zero-based contiguous  Inputs=5  DataPortForDefault=Additional data port  zeroidx=on  OutDataTypeStr=single  SaturateOnIntegerOverflow=off  InputSameDT=off
  Scope : Scope
  Sum of Elements1 : Sum  Inputs=+
  Switch : Switch  Criteria=u2 ~= 0  SaturateOnIntegerOverflow=off  InputSameDT=off
  Unit Delay : UnitDelay  SampleTime=-1  HasFrameUpgradeWarning=on
  sigAvg : Outport  OutDataTypeStr=single
  wires:
  Constant1/1 -> MATLAB Function/2(num)
  [sigAvg] -> sigAvg/1
  Multiport Switch/1 -> [sigAvg]
  [siginSingle] -> Multiport Switch/2
  [sigAvgQuick] -> Multiport Switch/6
  [sigAvgSimple] -> Multiport Switch/5
  [sigAvgSortWithoutEdge] -> Multiport Switch/4
  [sigAvgSortedMid] -> Multiport Switch/3
  Constant/1 -> Multiport Switch/1
  [sigin] -> Multiport Switch/7
  [sigin] -> Data Type Conversion/1
  sigin/1 -> [sigin]
  MATLAB Function/1(mid) -> [sigAvgSortedMid]
  Unit Delay/1 -> Switch/3
  MATLAB Function/2(withoutEdge) -> [sigAvgSortWithoutEdge]
  Data Type Conversion/1 -> Scope/1, Data Store Write/1, [siginSingle]
  Counter Limited/1 -> Data Store Write/2, Compare To Constant/1
  Gain1/1 -> [sigAvgQuick], Switch/1
  Switch/1 -> Unit Delay/1, [sigAvgSimple]
  Compare To Constant/1 -> Switch/2
  Sum of Elements1/1 -> Gain1/1
  Data Store Read/1 -> Sum of Elements1/1, MATLAB Function/1(u)

== system SigProcessFinished/SigProcessSub/CLHB02001_Filter/AVG8 ==
  sigin : Inport
  Compare To Constant : simulink/Logic and Bit Operations/Compare To Constant  relop===  const=0  OutDataTypeStr=boolean
  Constant : Constant  Value=cClCddAdc_D_u8FilterType  OutDataTypeStr=uint8
  Constant1 : Constant  Value=cClCddAdc_D_u8RawValueNum  OutDataTypeStr=uint8
  Counter Limited : simulink/Sources/Counter Limited  uplimit=cClCddAdc_D_u8RawValueNum-1  tsamp=-1
  Data Store Memory : DataStoreMemory  DataStoreName=ModFlapFroRIFbRaw  ReadBeforeWriteMsg=warning  WriteAfterWriteMsg=warning  WriteAfterReadMsg=warning  ShowAdditionalParam=off  OutDataTypeStr=single  Dimensions=[1 20]
      settings: CopyFcn=set_param(gcbh,'ShowName','off');
  Data Store Read : DataStoreRead  DataStoreName=ModFlapFroRIFbRaw  IndexOptions=Index vector (dialog)  Indices=1  OutputSizes=1
  Data Store Write : DataStoreWrite  DataStoreName=ModFlapFroRIFbRaw  DataStoreElements=ModFlapFroRIFbRaw  EnableIndexing=on  IndexMode=Zero-based  IndexOptions=Index vector (port)  Indices=1  OutputSizes=1
  Data Type Conversion : DataTypeConversion  OutDataTypeStr=single  SaturateOnIntegerOverflow=off  RndMeth=Floor
  Gain1 : Gain  Gain=1/cClCddAdc_D_u8RawValueNum
  MATLAB Function : MATLAB Function  TreatAsAtomicUnit=on
  Multiport Switch : MultiPortSwitch  DataPortOrder=Zero-based contiguous  Inputs=5  DataPortForDefault=Additional data port  zeroidx=on  OutDataTypeStr=single  SaturateOnIntegerOverflow=off  InputSameDT=off
  Scope : Scope
  Sum of Elements1 : Sum  Inputs=+
  Switch : Switch  Criteria=u2 ~= 0  SaturateOnIntegerOverflow=off  InputSameDT=off
  Unit Delay : UnitDelay  SampleTime=-1  HasFrameUpgradeWarning=on
  sigAvg : Outport  OutDataTypeStr=single
  wires:
  Data Store Read/1 -> MATLAB Function/1(u), Sum of Elements1/1
  Sum of Elements1/1 -> Gain1/1
  Compare To Constant/1 -> Switch/2
  Switch/1 -> [sigAvgSimple], Unit Delay/1
  Gain1/1 -> Switch/1, [sigAvgQuick]
  Counter Limited/1 -> Compare To Constant/1, Data Store Write/2
  Data Type Conversion/1 -> [siginSingle], Data Store Write/1, Scope/1
  MATLAB Function/2(withoutEdge) -> [sigAvgSortWithoutEdge]
  Unit Delay/1 -> Switch/3
  MATLAB Function/1(mid) -> [sigAvgSortedMid]
  sigin/1 -> [sigin]
  [sigin] -> Data Type Conversion/1
  [sigin] -> Multiport Switch/7
  Constant/1 -> Multiport Switch/1
  [sigAvgSortedMid] -> Multiport Switch/3
  [sigAvgSortWithoutEdge] -> Multiport Switch/4
  [sigAvgSimple] -> Multiport Switch/5
  [sigAvgQuick] -> Multiport Switch/6
  [siginSingle] -> Multiport Switch/2
  Multiport Switch/1 -> [sigAvg]
  [sigAvg] -> sigAvg/1
  Constant1/1 -> MATLAB Function/2(num)

== system SigProcessFinished/SigProcessSub/CLHB02001_Filter/AVG9 ==
  sigin : Inport
  Compare To Constant : simulink/Logic and Bit Operations/Compare To Constant  relop===  const=0  OutDataTypeStr=boolean
  Constant : Constant  Value=cClCddAdc_D_u8FilterType  OutDataTypeStr=uint8
  Constant1 : Constant  Value=cClCddAdc_D_u8RawValueNum  OutDataTypeStr=uint8
  Counter Limited : simulink/Sources/Counter Limited  uplimit=cClCddAdc_D_u8RawValueNum-1  tsamp=-1
  Data Store Memory : DataStoreMemory  DataStoreName=AqsPinRaw  ReadBeforeWriteMsg=warning  WriteAfterWriteMsg=warning  WriteAfterReadMsg=warning  ShowAdditionalParam=off  OutDataTypeStr=single  Dimensions=[1 20]
      settings: CopyFcn=set_param(gcbh,'ShowName','off');
  Data Store Read : DataStoreRead  DataStoreName=AqsPinRaw  IndexOptions=Index vector (dialog)  Indices=1  OutputSizes=1
  Data Store Write : DataStoreWrite  DataStoreName=AqsPinRaw  DataStoreElements=AqsPinRaw  EnableIndexing=on  IndexMode=Zero-based  IndexOptions=Index vector (port)  Indices=1  OutputSizes=1
  Data Type Conversion : DataTypeConversion  OutDataTypeStr=single  SaturateOnIntegerOverflow=off  RndMeth=Floor
  Gain1 : Gain  Gain=1/cClCddAdc_D_u8RawValueNum
  MATLAB Function : MATLAB Function  TreatAsAtomicUnit=on
  Multiport Switch : MultiPortSwitch  DataPortOrder=Zero-based contiguous  Inputs=5  DataPortForDefault=Additional data port  zeroidx=on  OutDataTypeStr=single  SaturateOnIntegerOverflow=off  InputSameDT=off
  Scope : Scope
  Sum of Elements1 : Sum  Inputs=+
  Switch : Switch  Criteria=u2 ~= 0  SaturateOnIntegerOverflow=off  InputSameDT=off
  Unit Delay : UnitDelay  SampleTime=-1  HasFrameUpgradeWarning=on
  sigAvg : Outport  OutDataTypeStr=single
  wires:
  Constant1/1 -> MATLAB Function/2(num)
  [sigAvg] -> sigAvg/1
  Multiport Switch/1 -> [sigAvg]
  [siginSingle] -> Multiport Switch/2
  [sigAvgQuick] -> Multiport Switch/6
  [sigAvgSimple] -> Multiport Switch/5
  [sigAvgSortWithoutEdge] -> Multiport Switch/4
  [sigAvgSortedMid] -> Multiport Switch/3
  Constant/1 -> Multiport Switch/1
  [sigin] -> Multiport Switch/7
  [sigin] -> Data Type Conversion/1
  sigin/1 -> [sigin]
  MATLAB Function/1(mid) -> [sigAvgSortedMid]
  Unit Delay/1 -> Switch/3
  MATLAB Function/2(withoutEdge) -> [sigAvgSortWithoutEdge]
  Data Type Conversion/1 -> Scope/1, Data Store Write/1, [siginSingle]
  Counter Limited/1 -> Data Store Write/2, Compare To Constant/1
  Gain1/1 -> [sigAvgQuick], Switch/1
  Switch/1 -> Unit Delay/1, [sigAvgSimple]
  Compare To Constant/1 -> Switch/2
  Sum of Elements1/1 -> Gain1/1
  Data Store Read/1 -> Sum of Elements1/1, MATLAB Function/1(u)

== system SigProcessFinished/SigProcessSub/CLHB02001_Filter/AVG/CLHB02002_Ad2Volt ==
  ad : Inport
  Gain : Gain  Gain=5/cClCddAdc_D_u16ADNum
  volt : Outport
  wires:
  ad/1 -> Gain/1
  Gain/1 -> volt/1

== matlab function SigProcessFinished/SigProcessSub/CLHB02001_Filter/AVG1/MATLAB Function ==
  data: u input; mid output; withoutEdge output; num input

function [mid, withoutEdge] = fcn(u,num)
% 输入u: 待排序数组
% 输入num: 滤波个数，max is 20
n = num;
for i = 1:n-1
    for j = 1:n-i
        if u(j) > u(j+1)
            temp = u(j);
            u(j) = u(j+1);
            u(j+1) = temp;
        end
    end
end
sortedData = u;

mid = sortedData(ceil(num/2)); % 取中间值
withoutEdge = mean(sortedData(2:num-1));

== matlab function SigProcessFinished/SigProcessSub/CLHB02001_Filter/AVG10/MATLAB Function ==
  data: u input; mid output; withoutEdge output; num input

function [mid, withoutEdge] = fcn(u,num)
% 输入u: 待排序数组
% 输入num: 滤波个数，max is 20
n = num;
for i = 1:n-1
    for j = 1:n-i
        if u(j) > u(j+1)
            temp = u(j);
            u(j) = u(j+1);
            u(j+1) = temp;
        end
    end
end
sortedData = u;

mid = sortedData(ceil(num/2)); % 取中间值
withoutEdge = mean(sortedData(2:num-1));

== matlab function SigProcessFinished/SigProcessSub/CLHB02001_Filter/AVG/MATLAB Function ==
  data: u input; mid output; withoutEdge output; num input

function [mid, withoutEdge] = fcn(u,num)
% 输入u: 待排序数组
% 输入num: 滤波个数，max is 20
n = num;
for i = 1:n-1
    for j = 1:n-i
        if u(j) > u(j+1)
            temp = u(j);
            u(j) = u(j+1);
            u(j+1) = temp;
        end
    end
end
sortedData = u;

mid = sortedData(ceil(num/2)); % 取中间值
withoutEdge = mean(sortedData(2:num-1));

== matlab function SigProcessFinished/SigProcessSub/CLHB02001_Filter/AVG2/MATLAB Function ==
  data: u input; mid output; withoutEdge output; num input

function [mid, withoutEdge] = fcn(u,num)
% 输入u: 待排序数组
% 输入num: 滤波个数，max is 20
n = num;
for i = 1:n-1
    for j = 1:n-i
        if u(j) > u(j+1)
            temp = u(j);
            u(j) = u(j+1);
            u(j+1) = temp;
        end
    end
end
sortedData = u;

mid = sortedData(ceil(num/2)); % 取中间值
withoutEdge = mean(sortedData(2:num-1));

== matlab function SigProcessFinished/SigProcessSub/CLHB02001_Filter/AVG3/MATLAB Function ==
  data: u input; mid output; withoutEdge output; num input

function [mid, withoutEdge] = fcn(u,num)
% 输入u: 待排序数组
% 输入num: 滤波个数，max is 20
n = num;
for i = 1:n-1
    for j = 1:n-i
        if u(j) > u(j+1)
            temp = u(j);
            u(j) = u(j+1);
            u(j+1) = temp;
        end
    end
end
sortedData = u;

mid = sortedData(ceil(num/2)); % 取中间值
withoutEdge = mean(sortedData(2:num-1));

== matlab function SigProcessFinished/SigProcessSub/CLHB02001_Filter/AVG4/MATLAB Function ==
  data: u input; mid output; withoutEdge output; num input

function [mid, withoutEdge] = fcn(u,num)
% 输入u: 待排序数组
% 输入num: 滤波个数，max is 20
n = num;
for i = 1:n-1
    for j = 1:n-i
        if u(j) > u(j+1)
            temp = u(j);
            u(j) = u(j+1);
            u(j+1) = temp;
        end
    end
end
sortedData = u;

mid = sortedData(ceil(num/2)); % 取中间值
withoutEdge = mean(sortedData(2:num-1));
